simulink model "ControlCascada"  (R2019a)
settings: Solver=VariableStepAuto  StartTime=0.0  StopTime=3  RelTol=1e-3
values from neighbouring files (symbols this model uses):
  B = 0.396912508    [funcioT.m]
  J = 0.190764151    [funcioT.m]
  Ka = 2.70653716    [funcioT.m]
  Km = Ka    (= 2.70653716)    [funcioT.m]
  L = 1.5e-3    (= 0.0015)    [funcioT.m]
  R = 4.8    [funcioT.m]
libraries: simulink x9
settings Model: Creator=Sergio  LastModifiedBy=User
settings DataIOCC: ReturnWorkspaceOutputs=off
settings DebuggingCC: PregeneratedLibrarySubsystemCodeDiagnostic=none  ArithmeticOperatorsInVariantConditions=warning
settings SFSimCC: SimUseLocalCustomCode=off
settings RTWCC: RTWUseLocalCustomCode=off

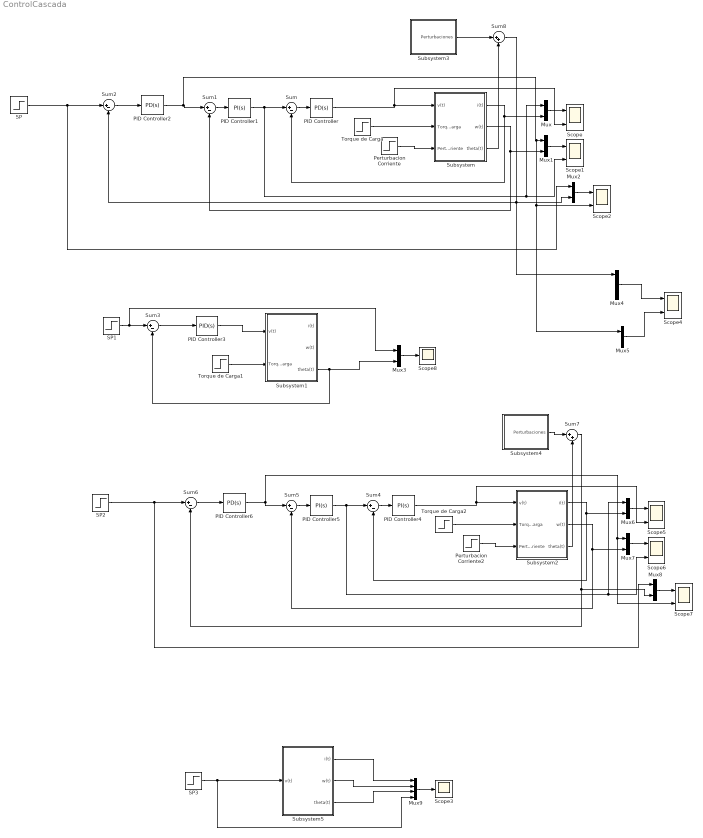
== system ControlCascada ==
  Mux{,1..3,5..8} (8 alike) : Mux  Inputs=2
  Mux4 : Mux  Inputs=3
  Mux9 : Mux
  PID Controller : simulink/Continuous/PID Controller  Controller=PD  Form=Parallel  TimeDomain=Continuous-time  SampleTime=-1  IntegratorMethod=Forward Euler  FilterMethod=Forward Euler  ControllerParametersSource=internal  P=3.6191162685072  I=0.000284403382998367  D=0.0177536521595203  UseFilter=on  N=36.2872486432421  TunerSelectOption=Transfer Function Based (PID Tuner App)  InitialConditionSource=internal  InitialConditionForIntegrator=0  InitialConditionForFilter=0  DifferentiatorICPrevScaledInput=0  ExternalReset=none  TrackingMode=off  Kt=1  LimitOutput=off  UpperSaturationLimit=inf  LowerSaturationLimit=-inf  LinearizeAsGain=on  AntiWindupMode=none  Kb=1  POutMin=[]  POutMax=[]  IOutMin=[]  IOutMax=[]  DOutMin=[]  DOutMax=[]  NOutMin=[]  NOutMax=[]  SumOutMin=[]  SumOutMax=[]  SaturationOutMin=[]  SaturationOutMax=[]  PParamMin=[]  PParamMax=[]  IParamMin=[]  IParamMax=[]  DParamMin=[]  DParamMax=[]  NParamMin=[]  NParamMax=[]  KbParamMin=[]  KbParamMax=[]  KtParamMin=[]  KtParamMax=[]  KbOutMin=[]  KbOutMax=[]  KtOutMin=[]  KtOutMax=[]  IntegratorOutMin=[]  IntegratorOutMax=[]  FilterOutMin=[]  FilterOutMax=[]  SumI1OutMin=[]  SumI1OutMax=[]  SumI2OutMin=[]  SumI2OutMax=[]  SumI3OutMin=[]  SumI3OutMax=[]  SumI4OutMin=[]  SumI4OutMax=[]  SumDOutMin=[]  SumDOutMax=[]  DifferentiatorOutMin=[]  DifferentiatorOutMax=[]  FilterDiffOutCoefMin=[]  FilterDiffOutCoefMax=[]  ReciprocalOutMin=[]  ReciprocalOutMax=[]  SumDenOutMin=[]  SumDenOutMax=[]  SumNumOutMin=[]  SumNumOutMax=[]  DivideOutMin=[]  DivideOutMax=[]  IntegratorContinuousStateAttributes=''  IntegratorStateMustResolveToSignalObject=off  IntegratorRTWStateStorageClass=Auto  FilterContinuousStateAttributes=''  FilterStateMustResolveToSignalObject=off  FilterRTWStateStorageClass=Auto  ParallelPVariant=InternalParameters  IdealPVariant=Disabled  IVariant=Disabled  DVariant=InternalParameters  IntegratorVariant=Disabled  SatVariant=Disabled  AWVariant=Disabled  PCopyVariant=Disabled  TRVariant=Disabled  FdbkBlocksVariant=Forward  IdealPFdbkVariant=Disabled  SatFdbkVariant=Disabled  DerivativeFilterVariant=ContFilter  NVariant=InternalParameters  NCopyVariant=Disabled  FilterICVariant=InternalICsFilter  IntegratorICVariant=Disabled  ExternalResetVariant=Disabled  TRSumVariant=Passthrough  SumFdbkVariant=Disabled  SumVariant=Sum_PD
  PID Controller1 : simulink/Continuous/PID Controller  Controller=PI  Form=Parallel  TimeDomain=Continuous-time  SampleTime=-1  IntegratorMethod=Forward Euler  FilterMethod=Forward Euler  ControllerParametersSource=internal  P=3.158554695701  I=6.43702288137936  D=-0.00136097830679664  UseFilter=on  N=1921.13300537321  TunerSelectOption=Transfer Function Based (PID Tuner App)  InitialConditionSource=internal  InitialConditionForIntegrator=0  InitialConditionForFilter=0  DifferentiatorICPrevScaledInput=0  ExternalReset=none  TrackingMode=off  Kt=1  LimitOutput=off  UpperSaturationLimit=inf  LowerSaturationLimit=-inf  LinearizeAsGain=on  AntiWindupMode=none  Kb=1  POutMin=[]  POutMax=[]  IOutMin=[]  IOutMax=[]  DOutMin=[]  DOutMax=[]  NOutMin=[]  NOutMax=[]  SumOutMin=[]  SumOutMax=[]  SaturationOutMin=[]  SaturationOutMax=[]  PParamMin=[]  PParamMax=[]  IParamMin=[]  IParamMax=[]  DParamMin=[]  DParamMax=[]  NParamMin=[]  NParamMax=[]  KbParamMin=[]  KbParamMax=[]  KtParamMin=[]  KtParamMax=[]  KbOutMin=[]  KbOutMax=[]  KtOutMin=[]  KtOutMax=[]  IntegratorOutMin=[]  IntegratorOutMax=[]  FilterOutMin=[]  FilterOutMax=[]  SumI1OutMin=[]  SumI1OutMax=[]  SumI2OutMin=[]  SumI2OutMax=[]  SumI3OutMin=[]  SumI3OutMax=[]  SumI4OutMin=[]  SumI4OutMax=[]  SumDOutMin=[]  SumDOutMax=[]  DifferentiatorOutMin=[]  DifferentiatorOutMax=[]  FilterDiffOutCoefMin=[]  FilterDiffOutCoefMax=[]  ReciprocalOutMin=[]  ReciprocalOutMax=[]  SumDenOutMin=[]  SumDenOutMax=[]  SumNumOutMin=[]  SumNumOutMax=[]  DivideOutMin=[]  DivideOutMax=[]  IntegratorContinuousStateAttributes=''  IntegratorStateMustResolveToSignalObject=off  IntegratorRTWStateStorageClass=Auto  FilterContinuousStateAttributes=''  FilterStateMustResolveToSignalObject=off  FilterRTWStateStorageClass=Auto  ParallelPVariant=InternalParameters  IdealPVariant=Disabled  IVariant=InternalParameters  DVariant=Disabled  IntegratorVariant=Continuous  SatVariant=Disabled  AWVariant=Passthrough  PCopyVariant=Disabled  TRVariant=Disabled  FdbkBlocksVariant=Forward  IdealPFdbkVariant=Disabled  SatFdbkVariant=Disabled  DerivativeFilterVariant=Disabled  NVariant=Disabled  NCopyVariant=Disabled_SignalSpec  FilterICVariant=Disabled  IntegratorICVariant=InternalICs  ExternalResetVariant=Disabled  TRSumVariant=Passthrough  SumFdbkVariant=Disabled  SumVariant=Sum_PI
  PID Controller2 : simulink/Continuous/PID Controller  Controller=PD  Form=Parallel  TimeDomain=Continuous-time  SampleTime=-1  IntegratorMethod=Forward Euler  FilterMethod=Forward Euler  ControllerParametersSource=internal  P=3.88889944431177  I=0.0290255889645778  D=0.401586761229223  UseFilter=on  N=6.36830270087834  TunerSelectOption=Transfer Function Based (PID Tuner App)  InitialConditionSource=internal  InitialConditionForIntegrator=0  InitialConditionForFilter=0  DifferentiatorICPrevScaledInput=0  ExternalReset=none  TrackingMode=off  Kt=1  LimitOutput=off  UpperSaturationLimit=inf  LowerSaturationLimit=-inf  LinearizeAsGain=on  AntiWindupMode=none  Kb=1  POutMin=[]  POutMax=[]  IOutMin=[]  IOutMax=[]  DOutMin=[]  DOutMax=[]  NOutMin=[]  NOutMax=[]  SumOutMin=[]  SumOutMax=[]  SaturationOutMin=[]  SaturationOutMax=[]  PParamMin=[]  PParamMax=[]  IParamMin=[]  IParamMax=[]  DParamMin=[]  DParamMax=[]  NParamMin=[]  NParamMax=[]  KbParamMin=[]  KbParamMax=[]  KtParamMin=[]  KtParamMax=[]  KbOutMin=[]  KbOutMax=[]  KtOutMin=[]  KtOutMax=[]  IntegratorOutMin=[]  IntegratorOutMax=[]  FilterOutMin=[]  FilterOutMax=[]  SumI1OutMin=[]  SumI1OutMax=[]  SumI2OutMin=[]  SumI2OutMax=[]  SumI3OutMin=[]  SumI3OutMax=[]  SumI4OutMin=[]  SumI4OutMax=[]  SumDOutMin=[]  SumDOutMax=[]  DifferentiatorOutMin=[]  DifferentiatorOutMax=[]  FilterDiffOutCoefMin=[]  FilterDiffOutCoefMax=[]  ReciprocalOutMin=[]  ReciprocalOutMax=[]  SumDenOutMin=[]  SumDenOutMax=[]  SumNumOutMin=[]  SumNumOutMax=[]  DivideOutMin=[]  DivideOutMax=[]  IntegratorContinuousStateAttributes=''  IntegratorStateMustResolveToSignalObject=off  IntegratorRTWStateStorageClass=Auto  FilterContinuousStateAttributes=''  FilterStateMustResolveToSignalObject=off  FilterRTWStateStorageClass=Auto  ParallelPVariant=InternalParameters  IdealPVariant=Disabled  IVariant=Disabled  DVariant=InternalParameters  IntegratorVariant=Disabled  SatVariant=Disabled  AWVariant=Disabled  PCopyVariant=Disabled  TRVariant=Disabled  FdbkBlocksVariant=Forward  IdealPFdbkVariant=Disabled  SatFdbkVariant=Disabled  DerivativeFilterVariant=ContFilter  NVariant=InternalParameters  NCopyVariant=Disabled  FilterICVariant=InternalICsFilter  IntegratorICVariant=Disabled  ExternalResetVariant=Disabled  TRSumVariant=Passthrough  SumFdbkVariant=Disabled  SumVariant=Sum_PD
  PID Controller3 : simulink/Continuous/PID Controller  Controller=PID  Form=Parallel  TimeDomain=Continuous-time  SampleTime=-1  IntegratorMethod=Forward Euler  FilterMethod=Forward Euler  ControllerParametersSource=internal  P=9.30783458507498  I=4.59103108664135  D=-0.0303242998985399  UseFilter=on  N=306.943098974006  TunerSelectOption=Transfer Function Based (PID Tuner App)  InitialConditionSource=internal  InitialConditionForIntegrator=0  InitialConditionForFilter=0  DifferentiatorICPrevScaledInput=0  ExternalReset=none  TrackingMode=off  Kt=1  LimitOutput=off  UpperSaturationLimit=inf  LowerSaturationLimit=-inf  LinearizeAsGain=on  AntiWindupMode=none  Kb=1  POutMin=[]  POutMax=[]  IOutMin=[]  IOutMax=[]  DOutMin=[]  DOutMax=[]  NOutMin=[]  NOutMax=[]  SumOutMin=[]  SumOutMax=[]  SaturationOutMin=[]  SaturationOutMax=[]  PParamMin=[]  PParamMax=[]  IParamMin=[]  IParamMax=[]  DParamMin=[]  DParamMax=[]  NParamMin=[]  NParamMax=[]  KbParamMin=[]  KbParamMax=[]  KtParamMin=[]  KtParamMax=[]  KbOutMin=[]  KbOutMax=[]  KtOutMin=[]  KtOutMax=[]  IntegratorOutMin=[]  IntegratorOutMax=[]  FilterOutMin=[]  FilterOutMax=[]  SumI1OutMin=[]  SumI1OutMax=[]  SumI2OutMin=[]  SumI2OutMax=[]  SumI3OutMin=[]  SumI3OutMax=[]  SumI4OutMin=[]  SumI4OutMax=[]  SumDOutMin=[]  SumDOutMax=[]  DifferentiatorOutMin=[]  DifferentiatorOutMax=[]  FilterDiffOutCoefMin=[]  FilterDiffOutCoefMax=[]  ReciprocalOutMin=[]  ReciprocalOutMax=[]  SumDenOutMin=[]  SumDenOutMax=[]  SumNumOutMin=[]  SumNumOutMax=[]  DivideOutMin=[]  DivideOutMax=[]  IntegratorContinuousStateAttributes=''  IntegratorStateMustResolveToSignalObject=off  IntegratorRTWStateStorageClass=Auto  FilterContinuousStateAttributes=''  FilterStateMustResolveToSignalObject=off  FilterRTWStateStorageClass=Auto  ParallelPVariant=InternalParameters  IdealPVariant=Disabled  IVariant=InternalParameters  DVariant=InternalParameters  IntegratorVariant=Continuous  SatVariant=Disabled  AWVariant=Passthrough  PCopyVariant=Disabled  TRVariant=Disabled  FdbkBlocksVariant=Forward  IdealPFdbkVariant=Disabled  SatFdbkVariant=Disabled  DerivativeFilterVariant=ContFilter  NVariant=InternalParameters  NCopyVariant=Disabled  FilterICVariant=InternalICsFilter  IntegratorICVariant=InternalICs  ExternalResetVariant=Disabled  TRSumVariant=Passthrough  SumFdbkVariant=Disabled  SumVariant=Sum_PID
  PID Controller4 : simulink/Continuous/PID Controller  Controller=PI  Form=Parallel  TimeDomain=Continuous-time  SampleTime=-1  IntegratorMethod=Forward Euler  FilterMethod=Forward Euler  ControllerParametersSource=internal  P=7.59332462474938  I=8.20113817301873  D=-0.740860787056165  UseFilter=on  N=10.2493272115558  TunerSelectOption=Transfer Function Based (PID Tuner App)  InitialConditionSource=internal  InitialConditionForIntegrator=0  InitialConditionForFilter=0  DifferentiatorICPrevScaledInput=0  ExternalReset=none  TrackingMode=off  Kt=1  LimitOutput=off  UpperSaturationLimit=inf  LowerSaturationLimit=-inf  LinearizeAsGain=on  AntiWindupMode=none  Kb=1  POutMin=[]  POutMax=[]  IOutMin=[]  IOutMax=[]  DOutMin=[]  DOutMax=[]  NOutMin=[]  NOutMax=[]  SumOutMin=[]  SumOutMax=[]  SaturationOutMin=[]  SaturationOutMax=[]  PParamMin=[]  PParamMax=[]  IParamMin=[]  IParamMax=[]  DParamMin=[]  DParamMax=[]  NParamMin=[]  NParamMax=[]  KbParamMin=[]  KbParamMax=[]  KtParamMin=[]  KtParamMax=[]  KbOutMin=[]  KbOutMax=[]  KtOutMin=[]  KtOutMax=[]  IntegratorOutMin=[]  IntegratorOutMax=[]  FilterOutMin=[]  FilterOutMax=[]  SumI1OutMin=[]  SumI1OutMax=[]  SumI2OutMin=[]  SumI2OutMax=[]  SumI3OutMin=[]  SumI3OutMax=[]  SumI4OutMin=[]  SumI4OutMax=[]  SumDOutMin=[]  SumDOutMax=[]  DifferentiatorOutMin=[]  DifferentiatorOutMax=[]  FilterDiffOutCoefMin=[]  FilterDiffOutCoefMax=[]  ReciprocalOutMin=[]  ReciprocalOutMax=[]  SumDenOutMin=[]  SumDenOutMax=[]  SumNumOutMin=[]  SumNumOutMax=[]  DivideOutMin=[]  DivideOutMax=[]  IntegratorContinuousStateAttributes=''  IntegratorStateMustResolveToSignalObject=off  IntegratorRTWStateStorageClass=Auto  FilterContinuousStateAttributes=''  FilterStateMustResolveToSignalObject=off  FilterRTWStateStorageClass=Auto  ParallelPVariant=InternalParameters  IdealPVariant=Disabled  IVariant=InternalParameters  DVariant=Disabled  IntegratorVariant=Continuous  SatVariant=Disabled  AWVariant=Passthrough  PCopyVariant=Disabled  TRVariant=Disabled  FdbkBlocksVariant=Forward  IdealPFdbkVariant=Disabled  SatFdbkVariant=Disabled  DerivativeFilterVariant=Disabled  NVariant=Disabled  NCopyVariant=Disabled_SignalSpec  FilterICVariant=Disabled  IntegratorICVariant=InternalICs  ExternalResetVariant=Disabled  TRSumVariant=Passthrough  SumFdbkVariant=Disabled  SumVariant=Sum_PI
  PID Controller5 : simulink/Continuous/PID Controller  Controller=PI  Form=Parallel  TimeDomain=Continuous-time  SampleTime=-1  IntegratorMethod=Forward Euler  FilterMethod=Forward Euler  ControllerParametersSource=internal  P=4.71404322464436  I=3.2012603855784  D=-0.0636654254910309  UseFilter=on  N=74.0440072187763  TunerSelectOption=Transfer Function Based (PID Tuner App)  InitialConditionSource=internal  InitialConditionForIntegrator=0  InitialConditionForFilter=0  DifferentiatorICPrevScaledInput=0  ExternalReset=none  TrackingMode=off  Kt=1  LimitOutput=off  UpperSaturationLimit=inf  LowerSaturationLimit=-inf  LinearizeAsGain=on  AntiWindupMode=none  Kb=1  POutMin=[]  POutMax=[]  IOutMin=[]  IOutMax=[]  DOutMin=[]  DOutMax=[]  NOutMin=[]  NOutMax=[]  SumOutMin=[]  SumOutMax=[]  SaturationOutMin=[]  SaturationOutMax=[]  PParamMin=[]  PParamMax=[]  IParamMin=[]  IParamMax=[]  DParamMin=[]  DParamMax=[]  NParamMin=[]  NParamMax=[]  KbParamMin=[]  KbParamMax=[]  KtParamMin=[]  KtParamMax=[]  KbOutMin=[]  KbOutMax=[]  KtOutMin=[]  KtOutMax=[]  IntegratorOutMin=[]  IntegratorOutMax=[]  FilterOutMin=[]  FilterOutMax=[]  SumI1OutMin=[]  SumI1OutMax=[]  SumI2OutMin=[]  SumI2OutMax=[]  SumI3OutMin=[]  SumI3OutMax=[]  SumI4OutMin=[]  SumI4OutMax=[]  SumDOutMin=[]  SumDOutMax=[]  DifferentiatorOutMin=[]  DifferentiatorOutMax=[]  FilterDiffOutCoefMin=[]  FilterDiffOutCoefMax=[]  ReciprocalOutMin=[]  ReciprocalOutMax=[]  SumDenOutMin=[]  SumDenOutMax=[]  SumNumOutMin=[]  SumNumOutMax=[]  DivideOutMin=[]  DivideOutMax=[]  IntegratorContinuousStateAttributes=''  IntegratorStateMustResolveToSignalObject=off  IntegratorRTWStateStorageClass=Auto  FilterContinuousStateAttributes=''  FilterStateMustResolveToSignalObject=off  FilterRTWStateStorageClass=Auto  ParallelPVariant=InternalParameters  IdealPVariant=Disabled  IVariant=InternalParameters  DVariant=Disabled  IntegratorVariant=Continuous  SatVariant=Disabled  AWVariant=Passthrough  PCopyVariant=Disabled  TRVariant=Disabled  FdbkBlocksVariant=Forward  IdealPFdbkVariant=Disabled  SatFdbkVariant=Disabled  DerivativeFilterVariant=Disabled  NVariant=Disabled  NCopyVariant=Disabled_SignalSpec  FilterICVariant=Disabled  IntegratorICVariant=InternalICs  ExternalResetVariant=Disabled  TRSumVariant=Passthrough  SumFdbkVariant=Disabled  SumVariant=Sum_PI
  PID Controller6 : simulink/Continuous/PID Controller  Controller=PD  Form=Parallel  TimeDomain=Continuous-time  SampleTime=-1  IntegratorMethod=Forward Euler  FilterMethod=Forward Euler  ControllerParametersSource=internal  P=2.24463473851023  I=0.0290255889645778  D=0.603461767082069  UseFilter=on  N=4.59340174312184  TunerSelectOption=Transfer Function Based (PID Tuner App)  InitialConditionSource=internal  InitialConditionForIntegrator=0  InitialConditionForFilter=0  DifferentiatorICPrevScaledInput=0  ExternalReset=none  TrackingMode=off  Kt=1  LimitOutput=off  UpperSaturationLimit=inf  LowerSaturationLimit=-inf  LinearizeAsGain=on  AntiWindupMode=none  Kb=1  POutMin=[]  POutMax=[]  IOutMin=[]  IOutMax=[]  DOutMin=[]  DOutMax=[]  NOutMin=[]  NOutMax=[]  SumOutMin=[]  SumOutMax=[]  SaturationOutMin=[]  SaturationOutMax=[]  PParamMin=[]  PParamMax=[]  IParamMin=[]  IParamMax=[]  DParamMin=[]  DParamMax=[]  NParamMin=[]  NParamMax=[]  KbParamMin=[]  KbParamMax=[]  KtParamMin=[]  KtParamMax=[]  KbOutMin=[]  KbOutMax=[]  KtOutMin=[]  KtOutMax=[]  IntegratorOutMin=[]  IntegratorOutMax=[]  FilterOutMin=[]  FilterOutMax=[]  SumI1OutMin=[]  SumI1OutMax=[]  SumI2OutMin=[]  SumI2OutMax=[]  SumI3OutMin=[]  SumI3OutMax=[]  SumI4OutMin=[]  SumI4OutMax=[]  SumDOutMin=[]  SumDOutMax=[]  DifferentiatorOutMin=[]  DifferentiatorOutMax=[]  FilterDiffOutCoefMin=[]  FilterDiffOutCoefMax=[]  ReciprocalOutMin=[]  ReciprocalOutMax=[]  SumDenOutMin=[]  SumDenOutMax=[]  SumNumOutMin=[]  SumNumOutMax=[]  DivideOutMin=[]  DivideOutMax=[]  IntegratorContinuousStateAttributes=''  IntegratorStateMustResolveToSignalObject=off  IntegratorRTWStateStorageClass=Auto  FilterContinuousStateAttributes=''  FilterStateMustResolveToSignalObject=off  FilterRTWStateStorageClass=Auto  ParallelPVariant=InternalParameters  IdealPVariant=Disabled  IVariant=Disabled  DVariant=InternalParameters  IntegratorVariant=Disabled  SatVariant=Disabled  AWVariant=Disabled  PCopyVariant=Disabled  TRVariant=Disabled  FdbkBlocksVariant=Forward  IdealPFdbkVariant=Disabled  SatFdbkVariant=Disabled  DerivativeFilterVariant=ContFilter  NVariant=InternalParameters  NCopyVariant=Disabled  FilterICVariant=InternalICsFilter  IntegratorICVariant=Disabled  ExternalResetVariant=Disabled  TRSumVariant=Passthrough  SumFdbkVariant=Disabled  SumVariant=Sum_PD
  Perturbacion Corriente : Step  Time=15  After=2  SampleTime=0
  Perturbacion Corriente2 : Step  Time=15  After=2  SampleTime=0
  SP : Step  Time=2  After=0.5  SampleTime=0
  SP1 : Step  Time=0.5  After=0.588  SampleTime=0
  SP2 : Step  Time=2  After=0.5  SampleTime=0
  SP3 : Step  Time=0.5  After=12  SampleTime=0
  Scope{,1..2,4..7} (7 alike) : Scope  NumInputPorts=2
  Scope3 : Scope
  Scope8 : Scope
  Subsystem : Subsystem
  Subsystem1 : Subsystem
  Subsystem2 : Subsystem
  Subsystem3 : Subsystem
  Subsystem4 : Subsystem
  Subsystem5 : Subsystem
  Sum{,1..6} (7 alike) : Sum  Inputs=|+-
  Sum7 : Sum  Inputs=|++
  Sum8 : Sum  Inputs=|++
  Torque de Carga : Step  Time=10  After=0.5*J  SampleTime=0
  Torque de Carga1 : Step  Time=10  After=0.5  SampleTime=0
  Torque de Carga2 : Step  Time=10  After=0.9*J  SampleTime=0
  wires:
  Torque de Carga/1 -> Subsystem/2(Torque Carga)
  Mux/1 -> Scope/1
  SP/1 -> Sum2/1, Mux2/1
  Sum/1 -> PID Controller/1
  PID Controller/1 -> Scope/2, Subsystem/1(v(t))
  Subsystem/1(i(t)) -> Mux/2, Sum/2
  Sum1/1 -> PID Controller1/1
  PID Controller1/1 -> Mux/1, Scope1/2, Sum/1
  Subsystem/2(w(t)) -> Mux1/2, Sum1/2
  Mux1/1 -> Scope1/1
  Sum2/1 -> PID Controller2/1
  PID Controller2/1 -> Scope2/2, Mux5/1, Mux1/1, Sum1/1
  Mux2/1 -> Scope2/1
  PID Controller3/1 -> Subsystem1/1(v(t))
  Sum3/1 -> PID Controller3/1
  Torque de Carga1/1 -> Subsystem1/2(Torque Carga)
  Subsystem1/3(theta(t)) -> Mux3/2, Sum3/2
  SP1/1 -> Mux3/1, Sum3/1
  Mux3/1 -> Scope8/1
  Mux4/1 -> Scope4/1
  Mux5/1 -> Scope4/2
  Perturbacion Corriente/1 -> Subsystem/3(Perturbacion de corriente)
  Subsystem2/1(i(t)) -> Mux6/2, Sum4/2
  Mux7/1 -> Scope6/1
  Sum6/1 -> PID Controller6/1
  Perturbacion Corriente2/1 -> Subsystem2/3(Perturbacion de corriente)
  PID Controller4/1 -> Scope5/2, Subsystem2/1(v(t))
  Sum4/1 -> PID Controller4/1
  Subsystem2/2(w(t)) -> Mux7/2, Sum5/2
  SP2/1 -> Mux8/1, Sum6/1
  Mux6/1 -> Scope5/1
  PID Controller6/1 -> Scope7/2, Mux7/1, Sum5/1
  Torque de Carga2/1 -> Subsystem2/2(Torque Carga)
  PID Controller5/1 -> Mux6/1, Scope6/2, Sum4/1
  Mux8/1 -> Scope7/1
  Sum5/1 -> PID Controller5/1
  Subsystem4/1("Perturbaciones ") -> Sum7/1
  Subsystem2/3(theta(t)) -> Sum7/2
  Sum7/1 -> Sum6/2, Mux8/2
  Subsystem3/1("Perturbaciones ") -> Sum8/1
  Subsystem/3(theta(t)) -> Sum8/2
  Sum8/1 -> Mux4/1, Sum2/2, Mux2/2
  SP3/1 -> Mux9/4, Subsystem5/1(v(t))
  Mux9/1 -> Scope3/1
  Subsystem5/1(i(t)) -> Mux9/1
  Subsystem5/2(w(t)) -> Mux9/2
  Subsystem5/3(theta(t)) -> Mux9/3

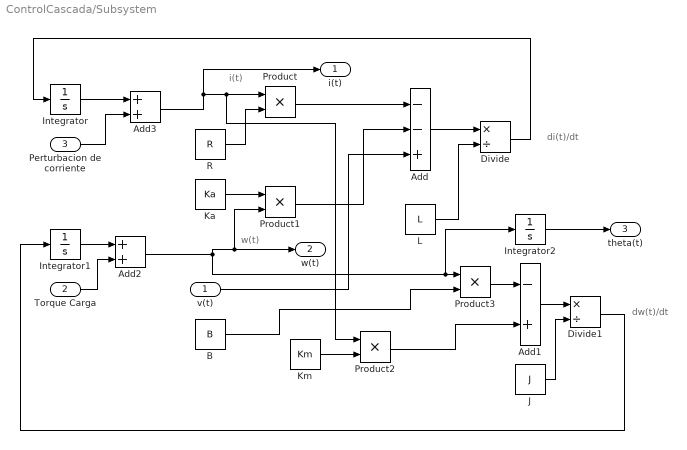
== system ControlCascada/Subsystem ==
  note: i(t)
  note: w(t)
  note: di(t)/dt
  note: dw(t)/dt
  v(t) : Inport
  Torque Carga : Inport  Port=2
  Perturbacion de corriente : Inport  Port=3
  Add : Sum  Inputs=--+
  Add1 : Sum  Inputs=-+
  Add2 : Sum
  Add3 : Sum
  B : Constant  Value=B
  Divide : Product  Inputs=*/
  Divide1 : Product  Inputs=*/
  Integrator : Integrator
  Integrator1 : Integrator
  Integrator2 : Integrator
  J : Constant  Value=J
  Ka : Constant  Value=Ka
  Km : Constant  Value=Km
  L : Constant  Value=L
  Product{,1..3} (4 alike) : Product
  R : Constant  Value=R
  i(t) : Outport
  w(t) : Outport  Port=2
  theta(t) : Outport  Port=3
  wires:
  v(t)/1 -> Add/3
  Divide1/1 -> Integrator1/1
  Product1/1 -> Add/2
  Product/1 -> Add/1
  Divide/1 -> Integrator/1
  Km/1 -> Product2/2
  L/1 -> Divide/2
  Add/1 -> Divide/1
  J/1 -> Divide1/2
  Product2/1 -> Add1/2
  B/1 -> Product3/2
  Integrator2/1 -> theta(t)/1
  Add1/1 -> Divide1/1
  Product3/1 -> Add1/1
  R/1 -> Product/2
  Ka/1 -> Product1/1
  Integrator1/1 -> Add2/1
  Add2/1 -> w(t)/1, Product1/2, Integrator2/1, Product3/1
  Torque Carga/1 -> Add2/2
  Add3/1 -> i(t)/1, Product2/1, Product/1
  Integrator/1 -> Add3/1
  Perturbacion de corriente/1 -> Add3/2

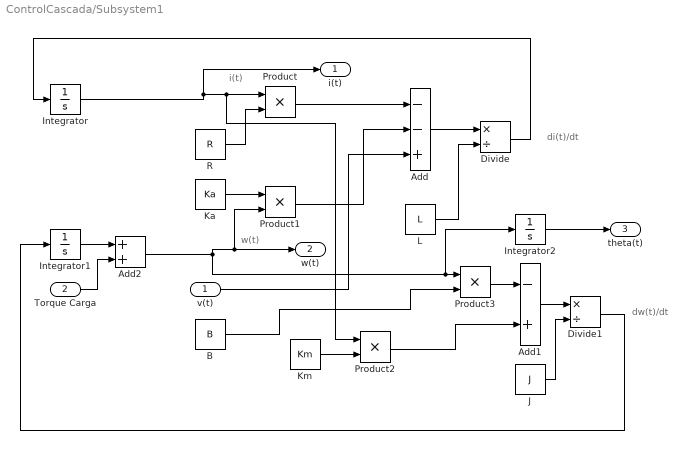
== system ControlCascada/Subsystem1 ==
  note: i(t)
  note: w(t)
  note: di(t)/dt
  note: dw(t)/dt
  v(t) : Inport
  Torque Carga : Inport  Port=2
  Add : Sum  Inputs=--+
  Add1 : Sum  Inputs=-+
  Add2 : Sum
  B : Constant  Value=B
  Divide : Product  Inputs=*/
  Divide1 : Product  Inputs=*/
  Integrator : Integrator
  Integrator1 : Integrator
  Integrator2 : Integrator
  J : Constant  Value=J
  Ka : Constant  Value=Ka
  Km : Constant  Value=Km
  L : Constant  Value=L
  Product{,1..3} (4 alike) : Product
  R : Constant  Value=R
  i(t) : Outport
  w(t) : Outport  Port=2
  theta(t) : Outport  Port=3
  wires:
  v(t)/1 -> Add/3
  Divide1/1 -> Integrator1/1
  Product1/1 -> Add/2
  Product/1 -> Add/1
  Divide/1 -> Integrator/1
  Km/1 -> Product2/2
  L/1 -> Divide/2
  Add/1 -> Divide/1
  J/1 -> Divide1/2
  Product2/1 -> Add1/2
  B/1 -> Product3/2
  Integrator2/1 -> theta(t)/1
  Add1/1 -> Divide1/1
  Product3/1 -> Add1/1
  R/1 -> Product/2
  Ka/1 -> Product1/1
  Integrator1/1 -> Add2/1
  Add2/1 -> w(t)/1, Product1/2, Integrator2/1, Product3/1
  Torque Carga/1 -> Add2/2
  Integrator/1 -> i(t)/1, Product2/1, Product/1

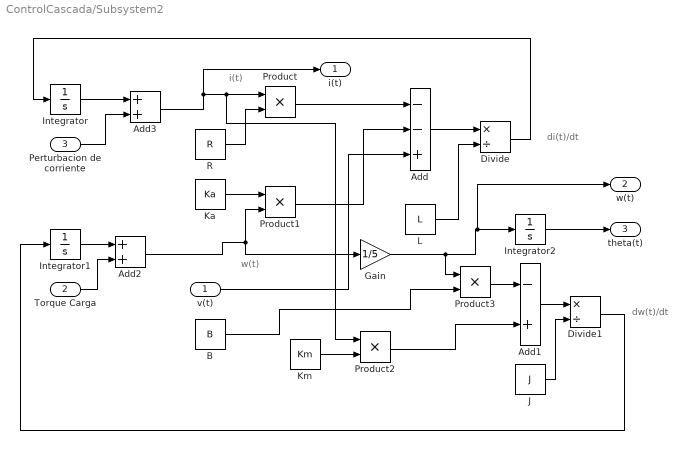
== system ControlCascada/Subsystem2 ==
  note: i(t)
  note: w(t)
  note: di(t)/dt
  note: dw(t)/dt
  v(t) : Inport
  Torque Carga : Inport  Port=2
  Perturbacion de corriente : Inport  Port=3
  Add : Sum  Inputs=--+
  Add1 : Sum  Inputs=-+
  Add2 : Sum
  Add3 : Sum
  B : Constant  Value=B
  Divide : Product  Inputs=*/
  Divide1 : Product  Inputs=*/
  Gain : Gain  Gain=1/5
  Integrator : Integrator
  Integrator1 : Integrator
  Integrator2 : Integrator
  J : Constant  Value=J
  Ka : Constant  Value=Ka
  Km : Constant  Value=Km
  L : Constant  Value=L
  Product{,1..3} (4 alike) : Product
  R : Constant  Value=R
  i(t) : Outport
  w(t) : Outport  Port=2
  theta(t) : Outport  Port=3
  wires:
  v(t)/1 -> Add/3
  Divide1/1 -> Integrator1/1
  Product1/1 -> Add/2
  Product/1 -> Add/1
  Divide/1 -> Integrator/1
  Km/1 -> Product2/2
  L/1 -> Divide/2
  Add/1 -> Divide/1
  J/1 -> Divide1/2
  Product2/1 -> Add1/2
  B/1 -> Product3/2
  Integrator2/1 -> theta(t)/1
  Add1/1 -> Divide1/1
  Product3/1 -> Add1/1
  R/1 -> Product/2
  Ka/1 -> Product1/1
  Integrator1/1 -> Add2/1
  Torque Carga/1 -> Add2/2
  Add3/1 -> i(t)/1, Product2/1, Product/1
  Integrator/1 -> Add3/1
  Perturbacion de corriente/1 -> Add3/2
  Add2/1 -> Product1/2, Gain/1
  Gain/1 -> Product3/1, w(t)/1, Integrator2/1

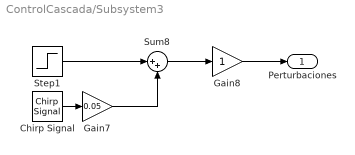
== system ControlCascada/Subsystem3 ==
  Chirp Signal : simulink/Sources/Chirp Signal  f1=1000  T=100  f2=1
  Gain7 : Gain  Gain=0.05
  Gain8 : Gain
  Step1 : Step  Time=40  SampleTime=0
  Sum8 : Sum  Inputs=|++
  "Perturbaciones " : Outport
  wires:
  Gain8/1 -> "Perturbaciones "/1
  Sum8/1 -> Gain8/1
  Gain7/1 -> Sum8/2
  Step1/1 -> Sum8/1
  Chirp Signal/1 -> Gain7/1

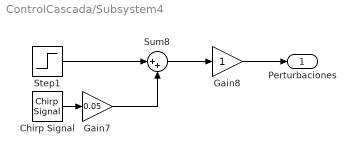
== system ControlCascada/Subsystem4 ==
  Chirp Signal : simulink/Sources/Chirp Signal  f1=100  T=100  f2=1
  Gain7 : Gain  Gain=0.05
  Gain8 : Gain
  Step1 : Step  Time=40  SampleTime=0
  Sum8 : Sum  Inputs=|++
  "Perturbaciones " : Outport
  wires:
  Gain8/1 -> "Perturbaciones "/1
  Sum8/1 -> Gain8/1
  Gain7/1 -> Sum8/2
  Step1/1 -> Sum8/1
  Chirp Signal/1 -> Gain7/1

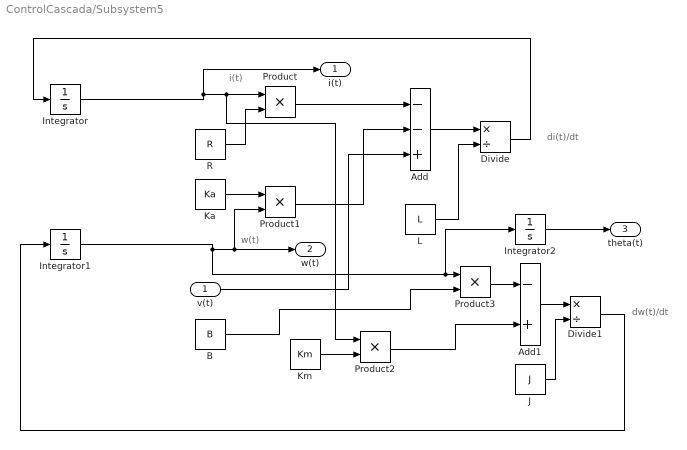
== system ControlCascada/Subsystem5 ==
  note: i(t)
  note: w(t)
  note: di(t)/dt
  note: dw(t)/dt
  v(t) : Inport
  Add : Sum  Inputs=--+
  Add1 : Sum  Inputs=-+
  B : Constant  Value=B
  Divide : Product  Inputs=*/
  Divide1 : Product  Inputs=*/
  Integrator : Integrator
  Integrator1 : Integrator
  Integrator2 : Integrator
  J : Constant  Value=J
  Ka : Constant  Value=Ka
  Km : Constant  Value=Km
  L : Constant  Value=L
  Product{,1..3} (4 alike) : Product
  R : Constant  Value=R
  i(t) : Outport
  w(t) : Outport  Port=2
  theta(t) : Outport  Port=3
  wires:
  v(t)/1 -> Add/3
  Divide1/1 -> Integrator1/1
  Product1/1 -> Add/2
  Product/1 -> Add/1
  Divide/1 -> Integrator/1
  Km/1 -> Product2/2
  L/1 -> Divide/2
  Add/1 -> Divide/1
  J/1 -> Divide1/2
  Product2/1 -> Add1/2
  B/1 -> Product3/2
  Integrator2/1 -> theta(t)/1
  Add1/1 -> Divide1/1
  Product3/1 -> Add1/1
  R/1 -> Product/2
  Ka/1 -> Product1/1
  Integrator1/1 -> Integrator2/1, Product3/1, w(t)/1, Product1/2
  Integrator/1 -> i(t)/1, Product2/1, Product/1
